simulink model "flightControlSystem"  (R2024a)
settings: Solver=ode3  StartTime=0  StopTime=TFinal  FixedStep=Ts  RelTol=1e-3  EnableMultiTasking=on
undefined symbols (not defined in the file): codertarget, Controller, DiscIntNeverNeededParam, Discrete, Estimator, g, gray, init, orient_ref, pos_ref, Sensors, Time, Ts, var_acc_angle_N, var_bias_gyr_N, var_gyro_p_N, Vehicle
libraries: simulink x37, slpidlib x4, ctrlSharedLib x4, sharedtransform x3, parrotlib x1
(part 3 of 3)

== matlab function flightControlSystem/Control System/Path Planning/MATLAB Function2 ==
  data: image input; isGap output; gap output
function [isGap, gap] = checkRedRegionsGap(image)
    % checkRedRegionsGap checks if there is a gap between two red regions in an image.
    %
    % Inputs:
    %   - img: The input image (RGB format)
    %
    % Outputs:
    %   - isGap: Boolean value (true if there is a gap, false if not)
    %   - gap: The pixel distance of the gap (0 if no gap)
    
    % Convert the image to HSV color space
    hsv_img = rgb2hsv(image);

    % Define thresholds for red color in HSV space
    lower_red1 = [0, 0.5, 0.5];  % Lower bound for red hue
    upper_red1 = [0.05, 1, 1];   % Upper bound for red hue
    lower_red2 = [0.95, 0.5, 0.5]; % Lower bound for red hue (for hue wrap around)
    upper_red2 = [1, 1, 1];      % Upper bound for red hue (for hue wrap around)

    % Create a binary mask for red regions
    mask1 = (hsv_img(:,:,1) >= lower_red1(1) & hsv_img(:,:,1) <= upper_red1(1)) & ...
            (hsv_img(:,:,2) >= lower_red1(2) & hsv_img(:,:,2) <= upper_red1(2)) & ...
            (hsv_img(:,:,3) >= lower_red1(3) & hsv_img(:,:,3) <= upper_red1(3));

    mask2 = (hsv_img(:,:,1) >= lower_red2(1) & hsv_img(:,:,1) <= upper_red2(1)) & ...
            (hsv_img(:,:,2) >= lower_red2(2) & hsv_img(:,:,2) <= upper_red2(2)) & ...
            (hsv_img(:,:,3) >= lower_red2(3) & hsv_img(:,:,3) <= upper_red2(3));

    red_mask = mask1 | mask2;

    % Label connected components in the binary mask
    cc = bwconncomp(red_mask);

    % Number of connected red regions
    num_red_regions = cc.NumObjects;

    % Initialize output variables
    isGap = false;
    gap = 0;

    % Check if there are exactly two red regions
    if num_red_regions == 2
        % Extract the bounding boxes of the two regions
        stats = regionprops(cc, 'BoundingBox');

        % Calculate the gap between the two bounding boxes
        bb1 = stats(1).BoundingBox;
        bb2 = stats(2).BoundingBox;

        % Determine if there is a gap
        x1 = bb1(1) + bb1(3);
        x2 = bb2(1);
        gap = abs(x2 - x1);

        if gap > 0
            isGap = true;
        else
            gap = 0;  % Ensure gap is zero if regions are touching
        end
    end
end

== matlab function flightControlSystem/Control System/Path Planning/MATLAB Function1 ==
  data: image input; redAreaPercentage output; redbottom output
function [redAreaPercentage,redbottom] = checkRedArea(image)
    % Assume the image is in RGB format
    % Get the dimensions of the image
    [height, width, ~] = size(image);
    
    % Define the boundary width (e.g., 5% of the image dimensions)
    boundaryWidth = round( width * 0.5);
    
    % Extract the boundary regions (top, bottom, left, right)
    topBoundary = image(1:boundaryWidth, :, :);
    bottomBoundary = image(end-boundaryWidth+1:end, :, :);
    leftBoundary = image(:, 1:boundaryWidth, :);
    rightBoundary = image(:, end-boundaryWidth+1:end, :);
    
    % Thresholds for red color
    redThreshold = 100;
    greenThreshold = 50;
    blueThreshold = 50;
    
    % Create red masks for each boundary region
    redMaskTop = topBoundary(:,:,1) > redThreshold & topBoundary(:,:,2) < greenThreshold & topBoundary(:,:,3) < blueThreshold;
    redMaskBottom = bottomBoundary(:,:,1) > redThreshold & bottomBoundary(:,:,2) < greenThreshold & bottomBoundary(:,:,3) < blueThreshold;
    redMaskLeft = leftBoundary(:,:,1) > redThreshold & leftBoundary(:,:,2) < greenThreshold & leftBoundary(:,:,3) < blueThreshold;
    redMaskRight = rightBoundary(:,:,1) > redThreshold & rightBoundary(:,:,2) < greenThreshold & rightBoundary(:,:,3) < blueThreshold;
    
    % Calculate the total number of red pixels in all boundaries
    totalRedPixels = sum(redMaskTop(:)) + sum(redMaskLeft(:)) + sum(redMaskRight(:));
    total2=sum(redMaskBottom(:));
    total2ac=numel(redMaskBottom);
    % Calculate the total number of pixels in all boundary regions
    totalBoundaryPixels = numel(redMaskTop)+ numel(redMaskLeft) + numel(redMaskRight);
    
    % Calculate the collective percentage of red area across all boundaries
    redAreaPercentage = totalRedPixels / totalBoundaryPixels;
    redbottom=total2/total2ac;
end

== stateflow chart flightControlSystem/Control System/Path Planning/Chart1 ==
  state counting
    entry:
    data=0;
  state output
    entry:
    data=isCircle;
    during:
    data=isCircle;
  (default) -> counting
  counting -> output : after(20,sec)
  data: data output; isCircle input
